simulink library "inp"  (Simulink 7.4)
settings: Solver=ode45  StartTime=0.0  StopTime=10.0  RelTol=1e-3
undefined symbols (not defined in the file): AINP_BrkPedalInterp_X_bar, C_TASK_10MS_S, ENUM_SHIFTER_D, ENUM_SHIFTER_N, ENUM_SHIFTER_P, ENUM_SHIFTER_R, KINP_BonnetCloseVehSpdThre_kph, KINP_EDUCoolantTempFilTm_s, KINP_EDUOilPressureFilTm_s, KINP_EDUOilTempFilTm_s, KINP_EDUSynchDisp_mm, KINP_EDUSynchPosnPWMDC_pct_LowerLimit, KINP_EDUSynchPosnPWMDC_pct_ovrdflg, KINP_EDUSynchPosnPWMDC_pct_ovrdval, KINP_EDUSynchPosnPWMDC_pct_UpperLimit, KINP_ShifterPosConfirmD_s, KINP_ShifterPosConfirmN_s, KINP_ShifterPosConfirmP_s, KINP_ShifterPosConfirmR_s, KINP_SingleAccPedalFltRateLim_pct, KINP_TMSpd2VehSpdSigNeg_rpm, KINP_TMSpd2VehSpdSigPos_rpm, KINP_ValidCheck_EDUSynchPosnPWMDC_dec, KINP_ValidCheck_EDUSynchPosnPWMDC_inc, KINP_ValidCheck_EDUSynchPosnPWMDC_lim, KINP_VehSpdSigKeepThres_kph, KPH2MPS, MIN2SEC, MINP_BrkPedalInterp_pct, MPS2KPH, PI, seat_version_control_block_callbacks, TIRE_RADIUS
libraries: inp_lib x166, hcu_lib x4, simulink x1
(part 2 of 9)

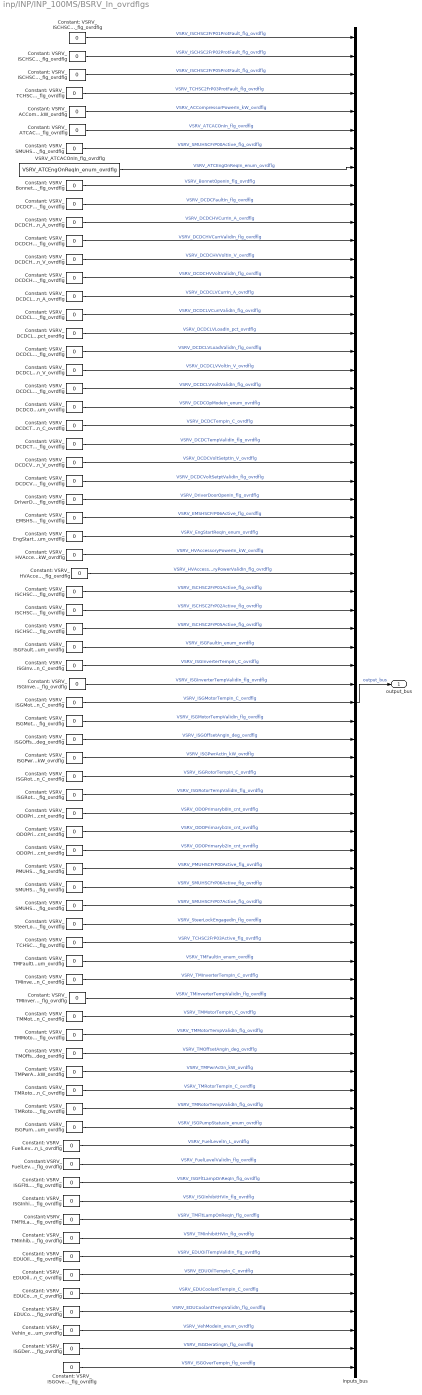
== system inp/INP/INP_100MS/BSRV_In_ovrdflgs ==
  Constant: VSRV_ACCompressorPowerIn_kW_ovrdflg : Constant  Value=0  OutDataTypeMode=boolean  OutDataTypeStr=boolean
  Constant: VSRV_ATCACOnIn_flg_ovrdflg : Constant  Value=0  OutDataTypeMode=boolean  OutDataTypeStr=boolean
  Constant: VSRV_BonnetOpenIn_flg_ovrdflg : Constant  Value=0  OutDataTypeMode=boolean  OutDataTypeStr=boolean
  Constant: VSRV_DCDCFaultIn_flg_ovrdflg : Constant  Value=0  OutDataTypeMode=boolean  OutDataTypeStr=boolean
  Constant: VSRV_DCDCHVCurrIn_A_ovrdflg : Constant  Value=0  OutDataTypeMode=boolean  OutDataTypeStr=boolean
  Constant: VSRV_DCDCHVCurrValidIn_flg_ovrdflg : Constant  Value=0  OutDataTypeMode=boolean  OutDataTypeStr=boolean
  Constant: VSRV_DCDCHVVoltIn_V_ovrdflg : Constant  Value=0  OutDataTypeMode=boolean  OutDataTypeStr=boolean
  Constant: VSRV_DCDCHVVoltValidIn_flg_ovrdflg : Constant  Value=0  OutDataTypeMode=boolean  OutDataTypeStr=boolean
  Constant: VSRV_DCDCLVCurrIn_A_ovrdflg : Constant  Value=0  OutDataTypeMode=boolean  OutDataTypeStr=boolean
  Constant: VSRV_DCDCLVCurrValidIn_flg_ovrdflg : Constant  Value=0  OutDataTypeMode=boolean  OutDataTypeStr=boolean
  Constant: VSRV_DCDCLVLoadIn_pct_ovrdflg : Constant  Value=0  OutDataTypeMode=boolean  OutDataTypeStr=boolean
  Constant: VSRV_DCDCLVLoadValidIn_flg_ovrdflg : Constant  Value=0  OutDataTypeMode=boolean  OutDataTypeStr=boolean
  Constant: VSRV_DCDCLVVoltIn_V_ovrdflg : Constant  Value=0  OutDataTypeMode=boolean  OutDataTypeStr=boolean
  Constant: VSRV_DCDCLVVoltValidIn_flg_ovrdflg : Constant  Value=0  OutDataTypeMode=boolean  OutDataTypeStr=boolean
  Constant: VSRV_DCDCOpModeIn_enum_ovrdflg : Constant  Value=0  OutDataTypeMode=boolean  OutDataTypeStr=boolean
  Constant: VSRV_DCDCTempIn_C_ovrdflg : Constant  Value=0  OutDataTypeMode=boolean  OutDataTypeStr=boolean
  Constant: VSRV_DCDCTempValidIn_flg_ovrdflg : Constant  Value=0  OutDataTypeMode=boolean  OutDataTypeStr=boolean
  Constant: VSRV_DCDCVoltSetptIn_V_ovrdflg : Constant  Value=0  OutDataTypeMode=boolean  OutDataTypeStr=boolean
  Constant: VSRV_DCDCVoltSetptValidIn_flg_ovrdflg : Constant  Value=0  OutDataTypeMode=boolean  OutDataTypeStr=boolean
  Constant: VSRV_DriverDoorOpenIn_flg_ovrdflg : Constant  Value=0  OutDataTypeMode=boolean  OutDataTypeStr=boolean
  Constant: VSRV_EDUCoolantTempIn_C_ovrdflg : Constant  Value=0  OutDataTypeMode=boolean  OutDataTypeStr=boolean
  Constant: VSRV_EDUCoolantTempValidIn_flg_ovrdflg : Constant  Value=0  OutDataTypeMode=boolean  OutDataTypeStr=boolean
  Constant: VSRV_EDUOilTempIn_C_ovrdflg : Constant  Value=0  OutDataTypeMode=boolean  OutDataTypeStr=boolean
  Constant: VSRV_EDUOilTempValidIn_flg_ovrdflg : Constant  Value=0  OutDataTypeMode=boolean  OutDataTypeStr=boolean
  Constant: VSRV_EMSHSCFrP06Active_flg_ovrdflg : Constant  Value=0  OutDataTypeMode=boolean  OutDataTypeStr=boolean
  Constant: VSRV_EngStartReqIn_enum_ovrdflg : Constant  Value=0  OutDataTypeMode=boolean  OutDataTypeStr=boolean
  Constant: VSRV_FuelLevelIn_L_ovrdflg : Constant  Value=0  OutDataTypeMode=boolean  OutDataTypeStr=boolean
  Constant: VSRV_HVAccessoryPowerIn_kW_ovrdflg : Constant  Value=0  OutDataTypeMode=boolean  OutDataTypeStr=boolean
  Constant: VSRV_HVAccessoryPowerValidIn_flg_ovrdflg : Constant  Value=0  OutDataTypeMode=boolean  OutDataTypeStr=boolean
  Constant: VSRV_ISCHSC2FrP01Active_flg_ovrdflg : Constant  Value=0  OutDataTypeMode=boolean  OutDataTypeStr=boolean
  Constant: VSRV_ISCHSC2FrP01ProtFault_flg_ovrdflg : Constant  Value=0  OutDataTypeMode=boolean  OutDataTypeStr=boolean
  Constant: VSRV_ISCHSC2FrP02Active_flg_ovrdflg : Constant  Value=0  OutDataTypeMode=boolean  OutDataTypeStr=boolean
  Constant: VSRV_ISCHSC2FrP02ProtFault_flg_ovrdflg : Constant  Value=0  OutDataTypeMode=boolean  OutDataTypeStr=boolean
  Constant: VSRV_ISCHSC2FrP05Active_flg_ovrdflg : Constant  Value=0  OutDataTypeMode=boolean  OutDataTypeStr=boolean
  Constant: VSRV_ISCHSC2FrP05ProtFault_flg_ovrdflg : Constant  Value=0  OutDataTypeMode=boolean  OutDataTypeStr=boolean
  Constant: VSRV_ISGDeratingIn_flg_ovrdflg : Constant  Value=0  OutDataTypeMode=boolean  OutDataTypeStr=boolean
  Constant: VSRV_ISGFaultIn_enum_ovrdflg : Constant  Value=0  OutDataTypeMode=boolean  OutDataTypeStr=boolean
  Constant: VSRV_ISGFltLampOnReqIn_flg_ovrdflg : Constant  Value=0  OutDataTypeMode=boolean  OutDataTypeStr=boolean
  Constant: VSRV_ISGInhibitHVIn_flg_ovrdflg : Constant  Value=0  OutDataTypeMode=boolean  OutDataTypeStr=boolean
  Constant: VSRV_ISGInverterTempIn_C_ovrdflg : Constant  Value=0  OutDataTypeMode=boolean  OutDataTypeStr=boolean
  Constant: VSRV_ISGInverterTempValidIn_flg_ovrdflg : Constant  Value=0  OutDataTypeMode=boolean  OutDataTypeStr=boolean
  Constant: VSRV_ISGMotorTempIn_C_ovrdflg : Constant  Value=0  OutDataTypeMode=boolean  OutDataTypeStr=boolean
  Constant: VSRV_ISGMotorTempValidIn_flg_ovrdflg : Constant  Value=0  OutDataTypeMode=boolean  OutDataTypeStr=boolean
  Constant: VSRV_ISGOffsetAngIn_deg_ovrdflg : Constant  Value=0  OutDataTypeMode=boolean  OutDataTypeStr=boolean
  Constant: VSRV_ISGOverTempIn_flg_ovrdflg : Constant  Value=0  OutDataTypeMode=boolean  OutDataTypeStr=boolean
  Constant: VSRV_ISGPumpStatusIn_enum_ovrdflg : Constant  Value=0  OutDataTypeMode=boolean  OutDataTypeStr=boolean
  Constant: VSRV_ISGPwrActIn_kW_ovrdflg : Constant  Value=0  OutDataTypeMode=boolean  OutDataTypeStr=boolean
  Constant: VSRV_ISGRotorTempIn_C_ovrdflg : Constant  Value=0  OutDataTypeMode=boolean  OutDataTypeStr=boolean
  Constant: VSRV_ISGRotorTempValidIn_flg_ovrdflg : Constant  Value=0  OutDataTypeMode=boolean  OutDataTypeStr=boolean
  Constant: VSRV_ODOPrimaryb0In_cnt_ovrdflg : Constant  Value=0  OutDataTypeMode=boolean  OutDataTypeStr=boolean
  Constant: VSRV_ODOPrimaryb1In_cnt_ovrdflg : Constant  Value=0  OutDataTypeMode=boolean  OutDataTypeStr=boolean
  Constant: VSRV_ODOPrimaryb2In_cnt_ovrdflg : Constant  Value=0  OutDataTypeMode=boolean  OutDataTypeStr=boolean
  Constant: VSRV_PMUHSCFrP00Active_flg_ovrdflg : Constant  Value=0  OutDataTypeMode=boolean  OutDataTypeStr=boolean
  Constant: VSRV_SMUHSCFrP00Active_flg_ovrdflg : Constant  Value=0  OutDataTypeMode=boolean  OutDataTypeStr=boolean
  Constant: VSRV_SMUHSCFrP06Active_flg_ovrdflg : Constant  Value=0  OutDataTypeMode=boolean  OutDataTypeStr=boolean
  Constant: VSRV_SMUHSCFrP07Active_flg_ovrdflg : Constant  Value=0  OutDataTypeMode=boolean  OutDataTypeStr=boolean
  Constant: VSRV_SteerLockEngagedIn_flg_ovrdflg : Constant  Value=0  OutDataTypeMode=boolean  OutDataTypeStr=boolean
  Constant: VSRV_TCHSC2FrP03Active_flg_ovrdflg : Constant  Value=0  OutDataTypeMode=boolean  OutDataTypeStr=boolean
  Constant: VSRV_TCHSC2FrP03ProtFault_flg_ovrdflg : Constant  Value=0  OutDataTypeMode=boolean  OutDataTypeStr=boolean
  Constant: VSRV_TMFaultIn_enum_ovrdflg : Constant  Value=0  OutDataTypeMode=boolean  OutDataTypeStr=boolean
  Constant: VSRV_TMInhibitHVIn_flg_ovrdflg : Constant  Value=0  OutDataTypeMode=boolean  OutDataTypeStr=boolean
  Constant: VSRV_TMInverterTempIn_C_ovrdflg : Constant  Value=0  OutDataTypeMode=boolean  OutDataTypeStr=boolean
  Constant: VSRV_TMInverterTempValidIn_flg_ovrdflg : Constant  Value=0  OutDataTypeMode=boolean  OutDataTypeStr=boolean
  Constant: VSRV_TMMotorTempIn_C_ovrdflg : Constant  Value=0  OutDataTypeMode=boolean  OutDataTypeStr=boolean
  Constant: VSRV_TMMotorTempValidIn_flg_ovrdflg : Constant  Value=0  OutDataTypeMode=boolean  OutDataTypeStr=boolean
  Constant: VSRV_TMOffsetAngIn_deg_ovrdflg : Constant  Value=0  OutDataTypeMode=boolean  OutDataTypeStr=boolean
  Constant: VSRV_TMPwrActIn_kW_ovrdflg : Constant  Value=0  OutDataTypeMode=boolean  OutDataTypeStr=boolean
  Constant: VSRV_TMRotorTempIn_C_ovrdflg : Constant  Value=0  OutDataTypeMode=boolean  OutDataTypeStr=boolean
  Constant: VSRV_TMRotorTempValidIn_flg_ovrdflg : Constant  Value=0  OutDataTypeMode=boolean  OutDataTypeStr=boolean
  Constant: VSRV_VehIn_enum_ovrdflg : Constant  Value=0  OutDataTypeMode=boolean  OutDataTypeStr=boolean
  Constant:VSRV_FuelLevelValidIn_flg_ovrdflg : Constant  Value=0  OutDataTypeMode=boolean  OutDataTypeStr=boolean
  Constant:VSRV_TMFltLampOnReqIn_flg_ovrdflg : Constant  Value=0  OutDataTypeMode=boolean  OutDataTypeStr=boolean
  VSRV_ATCACOnIn_flg_ovrdflg : DataStoreRead  DataStoreName=VSRV_ATCEngOnReqIn_enum_ovrdflg  SampleTime=-1
  inputs_bus : BusCreator  Inputs=73
  output_bus : Outport
  wires:
  Constant: VSRV_ISGOverTempIn_flg_ovrdflg/1 -> inputs_bus/73  "VSRV_ISGOverTempIn_flg_ovrdflg"
  Constant: VSRV_ISGDeratingIn_flg_ovrdflg/1 -> inputs_bus/72  "VSRV_ISGDeratingIn_flg_ovrdflg"
  Constant: VSRV_VehIn_enum_ovrdflg/1 -> inputs_bus/71  "VSRV_VehModeIn_enum_ovrdflg"
  Constant: VSRV_EDUCoolantTempValidIn_flg_ovrdflg/1 -> inputs_bus/70  "VSRV_EDUCoolantTempValidIn_flg_ovrdflg"
  Constant: VSRV_EDUCoolantTempIn_C_ovrdflg/1 -> inputs_bus/69  "VSRV_EDUCoolantTempIn_C_ovrdflg"
  Constant: VSRV_EDUOilTempIn_C_ovrdflg/1 -> inputs_bus/68  "VSRV_EDUOilTempIn_C_ovrdflg"
  Constant: VSRV_EDUOilTempValidIn_flg_ovrdflg/1 -> inputs_bus/67  "VSRV_EDUOilTempValidIn_flg_ovrdflg"
  Constant: VSRV_TMInhibitHVIn_flg_ovrdflg/1 -> inputs_bus/66  "VSRV_TMInhibitHVIn_flg_ovrdflg"
  Constant:VSRV_TMFltLampOnReqIn_flg_ovrdflg/1 -> inputs_bus/65  "VSRV_TMFltLampOnReqIn_flg_ovrdflg"
  Constant: VSRV_ISGInhibitHVIn_flg_ovrdflg/1 -> inputs_bus/64  "VSRV_ISGInhibitHVIn_flg_ovrdflg"
  Constant: VSRV_ISGFltLampOnReqIn_flg_ovrdflg/1 -> inputs_bus/63  "VSRV_ISGFltLampOnReqIn_flg_ovrdflg"
  Constant:VSRV_FuelLevelValidIn_flg_ovrdflg/1 -> inputs_bus/62  "VSRV_FuelLevelValidIn_flg_ovrdflg"
  Constant: VSRV_FuelLevelIn_L_ovrdflg/1 -> inputs_bus/61  "VSRV_FuelLevelIn_L_ovrdflg"
  Constant: VSRV_ISGPumpStatusIn_enum_ovrdflg/1 -> inputs_bus/60  "VSRV_ISGPumpStatusIn_enum_ovrdflg"
  Constant: VSRV_TMRotorTempValidIn_flg_ovrdflg/1 -> inputs_bus/59  "VSRV_TMRotorTempValidIn_flg_ovrdflg"
  Constant: VSRV_TMRotorTempIn_C_ovrdflg/1 -> inputs_bus/58  "VSRV_TMRotorTempIn_C_ovrdflg"
  Constant: VSRV_TMPwrActIn_kW_ovrdflg/1 -> inputs_bus/57  "VSRV_TMPwrActIn_kW_ovrdflg"
  Constant: VSRV_TMOffsetAngIn_deg_ovrdflg/1 -> inputs_bus/56  "VSRV_TMOffsetAngIn_deg_ovrdflg"
  Constant: VSRV_TMMotorTempValidIn_flg_ovrdflg/1 -> inputs_bus/55  "VSRV_TMMotorTempValidIn_flg_ovrdflg"
  Constant: VSRV_TMMotorTempIn_C_ovrdflg/1 -> inputs_bus/54  "VSRV_TMMotorTempIn_C_ovrdflg"
  Constant: VSRV_TMInverterTempValidIn_flg_ovrdflg/1 -> inputs_bus/53  "VSRV_TMInverterTempValidIn_flg_ovrdflg"
  Constant: VSRV_TMInverterTempIn_C_ovrdflg/1 -> inputs_bus/52  "VSRV_TMInverterTempIn_C_ovrdflg"
  Constant: VSRV_TMFaultIn_enum_ovrdflg/1 -> inputs_bus/51  "VSRV_TMFaultIn_enum_ovrdflg"
  Constant: VSRV_TCHSC2FrP03Active_flg_ovrdflg/1 -> inputs_bus/50  "VSRV_TCHSC2FrP03Active_flg_ovrdflg"
  Constant: VSRV_SteerLockEngagedIn_flg_ovrdflg/1 -> inputs_bus/49  "VSRV_SteerLockEngagedIn_flg_ovrdflg"
  Constant: VSRV_SMUHSCFrP07Active_flg_ovrdflg/1 -> inputs_bus/48  "VSRV_SMUHSCFrP07Active_flg_ovrdflg"
  Constant: VSRV_SMUHSCFrP06Active_flg_ovrdflg/1 -> inputs_bus/47  "VSRV_SMUHSCFrP06Active_flg_ovrdflg"
  Constant: VSRV_PMUHSCFrP00Active_flg_ovrdflg/1 -> inputs_bus/46  "VSRV_PMUHSCFrP00Active_flg_ovrdflg"
  Constant: VSRV_ODOPrimaryb2In_cnt_ovrdflg/1 -> inputs_bus/45  "VSRV_ODOPrimaryb2In_cnt_ovrdflg"
  Constant: VSRV_ODOPrimaryb1In_cnt_ovrdflg/1 -> inputs_bus/44  "VSRV_ODOPrimaryb1In_cnt_ovrdflg"
  Constant: VSRV_ODOPrimaryb0In_cnt_ovrdflg/1 -> inputs_bus/43  "VSRV_ODOPrimaryb0In_cnt_ovrdflg"
  Constant: VSRV_ISGRotorTempValidIn_flg_ovrdflg/1 -> inputs_bus/42  "VSRV_ISGRotorTempValidIn_flg_ovrdflg"
  Constant: VSRV_ISGRotorTempIn_C_ovrdflg/1 -> inputs_bus/41  "VSRV_ISGRotorTempIn_C_ovrdflg"
  Constant: VSRV_ISGPwrActIn_kW_ovrdflg/1 -> inputs_bus/40  "VSRV_ISGPwrActIn_kW_ovrdflg"
  Constant: VSRV_ISGOffsetAngIn_deg_ovrdflg/1 -> inputs_bus/39  "VSRV_ISGOffsetAngIn_deg_ovrdflg"
  Constant: VSRV_ISGMotorTempValidIn_flg_ovrdflg/1 -> inputs_bus/38  "VSRV_ISGMotorTempValidIn_flg_ovrdflg"
  Constant: VSRV_ISGMotorTempIn_C_ovrdflg/1 -> inputs_bus/37  "VSRV_ISGMotorTempIn_C_ovrdflg"
  Constant: VSRV_ISGInverterTempValidIn_flg_ovrdflg/1 -> inputs_bus/36  "VSRV_ISGInverterTempValidIn_flg_ovrdflg"
  Constant: VSRV_ISGInverterTempIn_C_ovrdflg/1 -> inputs_bus/35  "VSRV_ISGInverterTempIn_C_ovrdflg"
  Constant: VSRV_ISGFaultIn_enum_ovrdflg/1 -> inputs_bus/34  "VSRV_ISGFaultIn_enum_ovrdflg"
  Constant: VSRV_ISCHSC2FrP05Active_flg_ovrdflg/1 -> inputs_bus/33  "VSRV_ISCHSC2FrP05Active_flg_ovrdflg"
  Constant: VSRV_ISCHSC2FrP02Active_flg_ovrdflg/1 -> inputs_bus/32  "VSRV_ISCHSC2FrP02Active_flg_ovrdflg"
  Constant: VSRV_ISCHSC2FrP01Active_flg_ovrdflg/1 -> inputs_bus/31  "VSRV_ISCHSC2FrP01Active_flg_ovrdflg"
  Constant: VSRV_HVAccessoryPowerValidIn_flg_ovrdflg/1 -> inputs_bus/30  "VSRV_HVAccessoryPowerValidIn_flg_ovrdflg"
  Constant: VSRV_HVAccessoryPowerIn_kW_ovrdflg/1 -> inputs_bus/29  "VSRV_HVAccessoryPowerIn_kW_ovrdflg"
  Constant: VSRV_EngStartReqIn_enum_ovrdflg/1 -> inputs_bus/28  "VSRV_EngStartReqIn_enum_ovrdflg"
  Constant: VSRV_EMSHSCFrP06Active_flg_ovrdflg/1 -> inputs_bus/27  "VSRV_EMSHSCFrP06Active_flg_ovrdflg"
  Constant: VSRV_DriverDoorOpenIn_flg_ovrdflg/1 -> inputs_bus/26  "VSRV_DriverDoorOpenIn_flg_ovrdflg"
  Constant: VSRV_DCDCVoltSetptValidIn_flg_ovrdflg/1 -> inputs_bus/25  "VSRV_DCDCVoltSetptValidIn_flg_ovrdflg"
  Constant: VSRV_DCDCVoltSetptIn_V_ovrdflg/1 -> inputs_bus/24  "VSRV_DCDCVoltSetptIn_V_ovrdflg"
  Constant: VSRV_DCDCTempValidIn_flg_ovrdflg/1 -> inputs_bus/23  "VSRV_DCDCTempValidIn_flg_ovrdflg"
  Constant: VSRV_DCDCTempIn_C_ovrdflg/1 -> inputs_bus/22  "VSRV_DCDCTempIn_C_ovrdflg"
  Constant: VSRV_DCDCOpModeIn_enum_ovrdflg/1 -> inputs_bus/21  "VSRV_DCDCOpModeIn_enum_ovrdflg"
  Constant: VSRV_DCDCLVVoltValidIn_flg_ovrdflg/1 -> inputs_bus/20  "VSRV_DCDCLVVoltValidIn_flg_ovrdflg"
  Constant: VSRV_DCDCLVVoltIn_V_ovrdflg/1 -> inputs_bus/19  "VSRV_DCDCLVVoltIn_V_ovrdflg"
  Constant: VSRV_DCDCLVLoadValidIn_flg_ovrdflg/1 -> inputs_bus/18  "VSRV_DCDCLVLoadValidIn_flg_ovrdflg"
  Constant: VSRV_DCDCLVLoadIn_pct_ovrdflg/1 -> inputs_bus/17  "VSRV_DCDCLVLoadIn_pct_ovrdflg"
  Constant: VSRV_DCDCLVCurrValidIn_flg_ovrdflg/1 -> inputs_bus/16  "VSRV_DCDCLVCurrValidIn_flg_ovrdflg"
  Constant: VSRV_DCDCLVCurrIn_A_ovrdflg/1 -> inputs_bus/15  "VSRV_DCDCLVCurrIn_A_ovrdflg"
  Constant: VSRV_DCDCHVVoltValidIn_flg_ovrdflg/1 -> inputs_bus/14  "VSRV_DCDCHVVoltValidIn_flg_ovrdflg"
  Constant: VSRV_DCDCHVVoltIn_V_ovrdflg/1 -> inputs_bus/13  "VSRV_DCDCHVVoltIn_V_ovrdflg"
  Constant: VSRV_DCDCHVCurrValidIn_flg_ovrdflg/1 -> inputs_bus/12  "VSRV_DCDCHVCurrValidIn_flg_ovrdflg"
  Constant: VSRV_DCDCHVCurrIn_A_ovrdflg/1 -> inputs_bus/11  "VSRV_DCDCHVCurrIn_A_ovrdflg"
  Constant: VSRV_DCDCFaultIn_flg_ovrdflg/1 -> inputs_bus/10  "VSRV_DCDCFaultIn_flg_ovrdflg"
  Constant: VSRV_BonnetOpenIn_flg_ovrdflg/1 -> inputs_bus/9  "VSRV_BonnetOpenIn_flg_ovrdflg"
  VSRV_ATCACOnIn_flg_ovrdflg/1 -> inputs_bus/8  "VSRV_ATCEngOnReqIn_enum_ovrdflg"
  Constant: VSRV_SMUHSCFrP00Active_flg_ovrdflg/1 -> inputs_bus/7  "VSRV_SMUHSCFrP00Active_flg_ovrdflg"
  Constant: VSRV_ATCACOnIn_flg_ovrdflg/1 -> inputs_bus/6  "VSRV_ATCACOnIn_flg_ovrdflg"
  Constant: VSRV_ACCompressorPowerIn_kW_ovrdflg/1 -> inputs_bus/5  "VSRV_ACCompressorPowerIn_kW_ovrdflg"
  Constant: VSRV_TCHSC2FrP03ProtFault_flg_ovrdflg/1 -> inputs_bus/4  "VSRV_TCHSC2FrP03ProtFault_flg_ovrdflg"
  Constant: VSRV_ISCHSC2FrP05ProtFault_flg_ovrdflg/1 -> inputs_bus/3  "VSRV_ISCHSC2FrP05ProtFault_flg_ovrdflg"
  Constant: VSRV_ISCHSC2FrP02ProtFault_flg_ovrdflg/1 -> inputs_bus/2  "VSRV_ISCHSC2FrP02ProtFault_flg_ovrdflg"
  Constant: VSRV_ISCHSC2FrP01ProtFault_flg_ovrdflg/1 -> inputs_bus/1  "VSRV_ISCHSC2FrP01ProtFault_flg_ovrdflg"
  inputs_bus/1 -> output_bus/1  "output_bus"

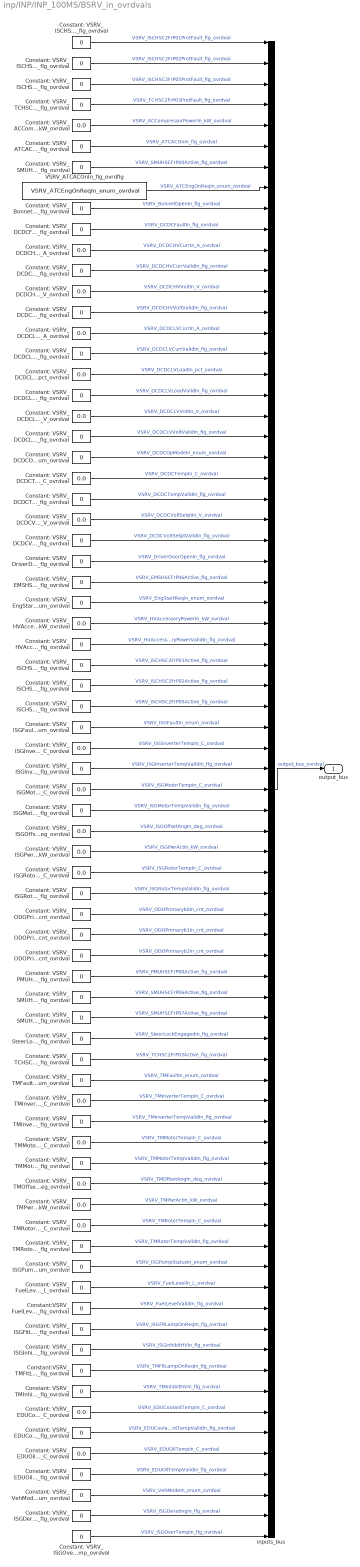
== system inp/INP/INP_100MS/BSRV_in_ovrdvals ==
  Constant: VSRV_ACCompressorPowerIn_kW_ovrdval : Constant  Value=0.0  OutDataTypeMode=single  OutDataTypeStr=single
  Constant: VSRV_ATCACOnIn_flg_ovrdval : Constant  Value=0  OutDataTypeMode=boolean  OutDataTypeStr=boolean
  Constant: VSRV_BonnetOpenIn_flg_ovrdval : Constant  Value=0  OutDataTypeMode=boolean  OutDataTypeStr=boolean
  Constant: VSRV_DCDCFaultIn_flg_ovrdval : Constant  Value=0  OutDataTypeMode=boolean  OutDataTypeStr=boolean
  Constant: VSRV_DCDCHVCurrIn_A_ovrdval : Constant  Value=0.0  OutDataTypeMode=single  OutDataTypeStr=single
  Constant: VSRV_DCDCHVCurrValidIn_flg_ovrdval : Constant  Value=0  OutDataTypeMode=boolean  OutDataTypeStr=boolean
  Constant: VSRV_DCDCHVVoltIn_V_ovrdval : Constant  Value=0.0  OutDataTypeMode=single  OutDataTypeStr=single
  Constant: VSRV_DCDCHVVoltValidIn_flg_ovrdval : Constant  Value=0  OutDataTypeMode=boolean  OutDataTypeStr=boolean
  Constant: VSRV_DCDCLVCurrIn_A_ovrdval : Constant  Value=0.0  OutDataTypeMode=single  OutDataTypeStr=single
  Constant: VSRV_DCDCLVCurrValidIn_flg_ovrdval : Constant  Value=0  OutDataTypeMode=boolean  OutDataTypeStr=boolean
  Constant: VSRV_DCDCLVLoadIn_pct_ovrdval : Constant  Value=0.0  OutDataTypeMode=single  OutDataTypeStr=single
  Constant: VSRV_DCDCLVLoadValidIn_flg_ovrdval : Constant  Value=0  OutDataTypeMode=boolean  OutDataTypeStr=boolean
  Constant: VSRV_DCDCLVVoltIn_V_ovrdval : Constant  Value=0.0  OutDataTypeMode=single  OutDataTypeStr=single
  Constant: VSRV_DCDCLVVoltValidIn_flg_ovrdval : Constant  Value=0  OutDataTypeMode=boolean  OutDataTypeStr=boolean
  Constant: VSRV_DCDCOpModeIn_enum_ovrdval : Constant  Value=0  OutDataTypeMode=uint8  OutDataTypeStr=uint8
  Constant: VSRV_DCDCTempIn_C_ovrdval : Constant  Value=0.0  OutDataTypeMode=single  OutDataTypeStr=single
  Constant: VSRV_DCDCTempValidIn_flg_ovrdval : Constant  Value=0  OutDataTypeMode=boolean  OutDataTypeStr=boolean
  Constant: VSRV_DCDCVoltSetptIn_V_ovrdval : Constant  Value=0.0  OutDataTypeMode=single  OutDataTypeStr=single
  Constant: VSRV_DCDCVoltSetptValidIn_flg_ovrdval : Constant  Value=0  OutDataTypeMode=boolean  OutDataTypeStr=boolean
  Constant: VSRV_DriverDoorOpenIn_flg_ovrdval : Constant  Value=0  OutDataTypeMode=boolean  OutDataTypeStr=boolean
  Constant: VSRV_EDUCoolantTempIn_C_ovrdval : Constant  Value=0.0  OutDataTypeMode=single  OutDataTypeStr=single
  Constant: VSRV_EDUCoolantTempValidIn_flg_ovrdval : Constant  Value=0  OutDataTypeMode=boolean  OutDataTypeStr=boolean
  Constant: VSRV_EDUOilTempIn_C_ovrdval : Constant  Value=0.0  OutDataTypeMode=single  OutDataTypeStr=single
  Constant: VSRV_EDUOilTempValidIn_flg_ovrdval : Constant  Value=0  OutDataTypeMode=boolean  OutDataTypeStr=boolean
  Constant: VSRV_EMSHSCFrP06Active_flg_ovrdval : Constant  Value=0  OutDataTypeMode=boolean  OutDataTypeStr=boolean
  Constant: VSRV_EngStartReqIn_enum_ovrdval : Constant  Value=0  OutDataTypeMode=uint8  OutDataTypeStr=uint8
  Constant: VSRV_FuelLevelIn_L_ovrdval : Constant  Value=0  OutDataTypeMode=single  OutDataTypeStr=single
  Constant: VSRV_HVAccessoryPowerIn_kW_ovrdval : Constant  Value=0.0  OutDataTypeMode=single  OutDataTypeStr=single
  Constant: VSRV_HVAccessoryPowerValidIn_flg_ovrdval : Constant  Value=0  OutDataTypeMode=boolean  OutDataTypeStr=boolean
  Constant: VSRV_ISCHSC2FrP01Active_flg_ovrdval : Constant  Value=0  OutDataTypeMode=boolean  OutDataTypeStr=boolean
  Constant: VSRV_ISCHSC2FrP01ProtFault_flg_ovrdval : Constant  Value=0  OutDataTypeMode=boolean  OutDataTypeStr=boolean
  Constant: VSRV_ISCHSC2FrP02Active_flg_ovrdval : Constant  Value=0  OutDataTypeMode=boolean  OutDataTypeStr=boolean
  Constant: VSRV_ISCHSC2FrP02ProtFault_flg_ovrdval : Constant  Value=0  OutDataTypeMode=boolean  OutDataTypeStr=boolean
  Constant: VSRV_ISCHSC2FrP05Active_flg_ovrdval : Constant  Value=0  OutDataTypeMode=boolean  OutDataTypeStr=boolean
  Constant: VSRV_ISCHSC2FrP05ProtFault_flg_ovrdval : Constant  Value=0  OutDataTypeMode=boolean  OutDataTypeStr=boolean
  Constant: VSRV_ISGDeratingIn_flg_ovrdval : Constant  Value=0  OutDataTypeMode=boolean  OutDataTypeStr=boolean
  Constant: VSRV_ISGFaultIn_enum_ovrdval : Constant  Value=0  OutDataTypeMode=uint8  OutDataTypeStr=uint8
  Constant: VSRV_ISGFltLampOnReqIn_flg_ovrdval : Constant  Value=0  OutDataTypeMode=boolean  OutDataTypeStr=boolean
  Constant: VSRV_ISGInhibitHVIn_flg_ovrdval : Constant  Value=0  OutDataTypeMode=boolean  OutDataTypeStr=boolean
  Constant: VSRV_ISGInverterTempIn_C_ovrdval : Constant  Value=0.0  OutDataTypeMode=single  OutDataTypeStr=single
  Constant: VSRV_ISGInverterTempValidIn_flg_ovrdval : Constant  Value=0  OutDataTypeMode=boolean  OutDataTypeStr=boolean
  Constant: VSRV_ISGMotorTempIn_C_ovrdval : Constant  Value=0.0  OutDataTypeMode=single  OutDataTypeStr=single
  Constant: VSRV_ISGMotorTempValidIn_flg_ovrdval : Constant  Value=0  OutDataTypeMode=boolean  OutDataTypeStr=boolean
  Constant: VSRV_ISGOffsetAngIn_deg_ovrdval : Constant  Value=0.0  OutDataTypeMode=single  OutDataTypeStr=single
  Constant: VSRV_ISGOverTemp_ovrdval : Constant  Value=0  OutDataTypeMode=boolean  OutDataTypeStr=boolean
  Constant: VSRV_ISGPumpStatusIn_enum_ovrdval : Constant  Value=0  OutDataTypeMode=uint8  OutDataTypeStr=uint8
  Constant: VSRV_ISGPwrActIn_kW_ovrdval : Constant  Value=0.0  OutDataTypeMode=single  OutDataTypeStr=single
  Constant: VSRV_ISGRotorTempIn_C_ovrdval : Constant  Value=0.0  OutDataTypeMode=single  OutDataTypeStr=single
  Constant: VSRV_ISGRotorTempValidIn_flg_ovrdval : Constant  Value=0  OutDataTypeMode=boolean  OutDataTypeStr=boolean
  Constant: VSRV_ODOPrimaryb0In_cnt_ovrdval : Constant  Value=0  OutDataTypeMode=uint8  OutDataTypeStr=uint8
  Constant: VSRV_ODOPrimaryb1In_cnt_ovrdval : Constant  Value=0  OutDataTypeMode=uint8  OutDataTypeStr=uint8
  Constant: VSRV_ODOPrimaryb2In_cnt_ovrdval : Constant  Value=0  OutDataTypeMode=uint8  OutDataTypeStr=uint8
  Constant: VSRV_PMUHSCFrP00Active_flg_ovrdval : Constant  Value=0  OutDataTypeMode=boolean  OutDataTypeStr=boolean
  Constant: VSRV_SMUHSCFrP00Active_flg_ovrdval : Constant  Value=0  OutDataTypeMode=boolean  OutDataTypeStr=boolean
  Constant: VSRV_SMUHSCFrP06Active_flg_ovrdval : Constant  Value=0  OutDataTypeMode=boolean  OutDataTypeStr=boolean
  Constant: VSRV_SMUHSCFrP07Active_flg_ovrdval : Constant  Value=0  OutDataTypeMode=boolean  OutDataTypeStr=boolean
  Constant: VSRV_SteerLockEngagedIn_flg_ovrdval : Constant  Value=0  OutDataTypeMode=boolean  OutDataTypeStr=boolean
  Constant: VSRV_TCHSC2FrP03Active_flg_ovrdval : Constant  Value=0  OutDataTypeMode=boolean  OutDataTypeStr=boolean
  Constant: VSRV_TCHSC2FrP03ProtFault_flg_ovrdval : Constant  Value=0  OutDataTypeMode=boolean  OutDataTypeStr=boolean
  Constant: VSRV_TMFaultIn_enum_ovrdval : Constant  Value=0  OutDataTypeMode=uint8  OutDataTypeStr=uint8
  Constant: VSRV_TMInhibitHVIn_flg_ovrdval : Constant  Value=0  OutDataTypeMode=boolean  OutDataTypeStr=boolean
  Constant: VSRV_TMInverterTempIn_C_ovrdval : Constant  Value=0.0  OutDataTypeMode=single  OutDataTypeStr=single
  Constant: VSRV_TMInverterTempValidIn_flg_ovrdval : Constant  Value=0  OutDataTypeMode=boolean  OutDataTypeStr=boolean
  Constant: VSRV_TMMotorTempIn_C_ovrdval : Constant  Value=0.0  OutDataTypeMode=single  OutDataTypeStr=single
  Constant: VSRV_TMMotorTempValidIn_flg_ovrdval : Constant  Value=0  OutDataTypeMode=boolean  OutDataTypeStr=boolean
  Constant: VSRV_TMOffsetAngIn_deg_ovrdval : Constant  Value=0.0  OutDataTypeMode=single  OutDataTypeStr=single
  Constant: VSRV_TMPwrActIn_kW_ovrdval : Constant  Value=0.0  OutDataTypeMode=single  OutDataTypeStr=single
  Constant: VSRV_TMRotorTempIn_C_ovrdval : Constant  Value=0.0  OutDataTypeMode=single  OutDataTypeStr=single
  Constant: VSRV_TMRotorTempValidIn_flg_ovrdval : Constant  Value=0  OutDataTypeMode=boolean  OutDataTypeStr=boolean
  Constant: VSRV_VehModeIn_enum_ovrdval : Constant  Value=0  OutDataTypeMode=uint8  OutDataTypeStr=uint8
  Constant:VSRV_FuelLevelValidIn_flg_ovrdval : Constant  Value=0  OutDataTypeMode=boolean  OutDataTypeStr=boolean
  Constant:VSRV_TMFltLampOnReqIn_flg_ovrdval : Constant  Value=0  OutDataTypeMode=boolean  OutDataTypeStr=boolean
  VSRV_ATCACOnIn_flg_ovrdflg : DataStoreRead  DataStoreName=VSRV_ATCEngOnReqIn_enum_ovrdval  SampleTime=-1
  inputs_bus : BusCreator  Inputs=73
  output_bus : Outport
  wires:
  Constant: VSRV_ISGOverTemp_ovrdval/1 -> inputs_bus/73  "VSRV_ISGOverTempIn_flg_ovrdval"
  Constant: VSRV_ISGDeratingIn_flg_ovrdval/1 -> inputs_bus/72  "VSRV_ISGDeratingIn_flg_ovrdval"
  Constant: VSRV_VehModeIn_enum_ovrdval/1 -> inputs_bus/71  "VSRV_VehModeIn_enum_ovrdval"
  Constant: VSRV_EDUOilTempValidIn_flg_ovrdval/1 -> inputs_bus/70  "VSRV_EDUOilTempValidIn_flg_ovrdval"
  Constant: VSRV_EDUOilTempIn_C_ovrdval/1 -> inputs_bus/69  "VSRV_EDUOilTempIn_C_ovrdval"
  Constant: VSRV_EDUCoolantTempValidIn_flg_ovrdval/1 -> inputs_bus/68  "VSRV_EDUCoolantTempValidIn_flg_ovrdval"
  Constant: VSRV_EDUCoolantTempIn_C_ovrdval/1 -> inputs_bus/67  "VSRV_EDUCoolantTempIn_C_ovrdval"
  Constant: VSRV_TMInhibitHVIn_flg_ovrdval/1 -> inputs_bus/66  "VSRV_TMInhibitHVIn_flg_ovrdval"
  Constant:VSRV_TMFltLampOnReqIn_flg_ovrdval/1 -> inputs_bus/65  "VSRV_TMFltLampOnReqIn_flg_ovrdval"
  Constant: VSRV_ISGInhibitHVIn_flg_ovrdval/1 -> inputs_bus/64  "VSRV_ISGInhibitHVIn_flg_ovrdval"
  Constant: VSRV_ISGFltLampOnReqIn_flg_ovrdval/1 -> inputs_bus/63  "VSRV_ISGFltLampOnReqIn_flg_ovrdval"
  Constant:VSRV_FuelLevelValidIn_flg_ovrdval/1 -> inputs_bus/62  "VSRV_FuelLevelValidIn_flg_ovrdval"
  Constant: VSRV_FuelLevelIn_L_ovrdval/1 -> inputs_bus/61  "VSRV_FuelLevelIn_L_ovrdval"
  Constant: VSRV_ISGPumpStatusIn_enum_ovrdval/1 -> inputs_bus/60  "VSRV_ISGPumpStatusIn_enum_ovrdval"
  Constant: VSRV_TMRotorTempValidIn_flg_ovrdval/1 -> inputs_bus/59  "VSRV_TMRotorTempValidIn_flg_ovrdval"
  Constant: VSRV_TMRotorTempIn_C_ovrdval/1 -> inputs_bus/58  "VSRV_TMRotorTempIn_C_ovrdval"
  Constant: VSRV_TMPwrActIn_kW_ovrdval/1 -> inputs_bus/57  "VSRV_TMPwrActIn_kW_ovrdval"
  Constant: VSRV_TMOffsetAngIn_deg_ovrdval/1 -> inputs_bus/56  "VSRV_TMOffsetAngIn_deg_ovrdval"
  Constant: VSRV_TMMotorTempValidIn_flg_ovrdval/1 -> inputs_bus/55  "VSRV_TMMotorTempValidIn_flg_ovrdval"
  Constant: VSRV_TMMotorTempIn_C_ovrdval/1 -> inputs_bus/54  "VSRV_TMMotorTempIn_C_ovrdval"
  Constant: VSRV_TMInverterTempValidIn_flg_ovrdval/1 -> inputs_bus/53  "VSRV_TMInverterTempValidIn_flg_ovrdval"
  Constant: VSRV_TMInverterTempIn_C_ovrdval/1 -> inputs_bus/52  "VSRV_TMInverterTempIn_C_ovrdval"
  Constant: VSRV_TMFaultIn_enum_ovrdval/1 -> inputs_bus/51  "VSRV_TMFaultIn_enum_ovrdval"
  Constant: VSRV_TCHSC2FrP03Active_flg_ovrdval/1 -> inputs_bus/50  "VSRV_TCHSC2FrP03Active_flg_ovrdval"
  Constant: VSRV_SteerLockEngagedIn_flg_ovrdval/1 -> inputs_bus/49  "VSRV_SteerLockEngagedIn_flg_ovrdval"
  Constant: VSRV_SMUHSCFrP07Active_flg_ovrdval/1 -> inputs_bus/48  "VSRV_SMUHSCFrP07Active_flg_ovrdval"
  Constant: VSRV_SMUHSCFrP06Active_flg_ovrdval/1 -> inputs_bus/47  "VSRV_SMUHSCFrP06Active_flg_ovrdval"
  Constant: VSRV_PMUHSCFrP00Active_flg_ovrdval/1 -> inputs_bus/46  "VSRV_PMUHSCFrP00Active_flg_ovrdval"
  Constant: VSRV_ODOPrimaryb2In_cnt_ovrdval/1 -> inputs_bus/45  "VSRV_ODOPrimaryb2In_cnt_ovrdval"
  Constant: VSRV_ODOPrimaryb1In_cnt_ovrdval/1 -> inputs_bus/44  "VSRV_ODOPrimaryb1In_cnt_ovrdval"
  Constant: VSRV_ODOPrimaryb0In_cnt_ovrdval/1 -> inputs_bus/43  "VSRV_ODOPrimaryb0In_cnt_ovrdval"
  Constant: VSRV_ISGRotorTempValidIn_flg_ovrdval/1 -> inputs_bus/42  "VSRV_ISGRotorTempValidIn_flg_ovrdval"
  Constant: VSRV_ISGRotorTempIn_C_ovrdval/1 -> inputs_bus/41  "VSRV_ISGRotorTempIn_C_ovrdval"
  Constant: VSRV_ISGPwrActIn_kW_ovrdval/1 -> inputs_bus/40  "VSRV_ISGPwrActIn_kW_ovrdval"
  Constant: VSRV_ISGOffsetAngIn_deg_ovrdval/1 -> inputs_bus/39  "VSRV_ISGOffsetAngIn_deg_ovrdval"
  Constant: VSRV_ISGMotorTempValidIn_flg_ovrdval/1 -> inputs_bus/38  "VSRV_ISGMotorTempValidIn_flg_ovrdval"
  Constant: VSRV_ISGMotorTempIn_C_ovrdval/1 -> inputs_bus/37  "VSRV_ISGMotorTempIn_C_ovrdval"
  Constant: VSRV_ISGInverterTempValidIn_flg_ovrdval/1 -> inputs_bus/36  "VSRV_ISGInverterTempValidIn_flg_ovrdval"
  Constant: VSRV_ISGInverterTempIn_C_ovrdval/1 -> inputs_bus/35  "VSRV_ISGInverterTempIn_C_ovrdval"
  Constant: VSRV_ISGFaultIn_enum_ovrdval/1 -> inputs_bus/34  "VSRV_ISGFaultIn_enum_ovrdval"
  Constant: VSRV_ISCHSC2FrP05Active_flg_ovrdval/1 -> inputs_bus/33  "VSRV_ISCHSC2FrP05Active_flg_ovrdval"
  Constant: VSRV_ISCHSC2FrP02Active_flg_ovrdval/1 -> inputs_bus/32  "VSRV_ISCHSC2FrP02Active_flg_ovrdval"
  Constant: VSRV_ISCHSC2FrP01Active_flg_ovrdval/1 -> inputs_bus/31  "VSRV_ISCHSC2FrP01Active_flg_ovrdval"
  Constant: VSRV_HVAccessoryPowerValidIn_flg_ovrdval/1 -> inputs_bus/30  "VSRV_HVAccessoryPowerValidIn_flg_ovrdval"
  Constant: VSRV_HVAccessoryPowerIn_kW_ovrdval/1 -> inputs_bus/29  "VSRV_HVAccessoryPowerIn_kW_ovrdval"
  Constant: VSRV_EngStartReqIn_enum_ovrdval/1 -> inputs_bus/28  "VSRV_EngStartReqIn_enum_ovrdval"
  Constant: VSRV_EMSHSCFrP06Active_flg_ovrdval/1 -> inputs_bus/27  "VSRV_EMSHSCFrP06Active_flg_ovrdval"
  Constant: VSRV_DriverDoorOpenIn_flg_ovrdval/1 -> inputs_bus/26  "VSRV_DriverDoorOpenIn_flg_ovrdval"
  Constant: VSRV_DCDCVoltSetptValidIn_flg_ovrdval/1 -> inputs_bus/25  "VSRV_DCDCVoltSetptValidIn_flg_ovrdval"
  Constant: VSRV_DCDCVoltSetptIn_V_ovrdval/1 -> inputs_bus/24  "VSRV_DCDCVoltSetptIn_V_ovrdval"
  Constant: VSRV_DCDCTempValidIn_flg_ovrdval/1 -> inputs_bus/23  "VSRV_DCDCTempValidIn_flg_ovrdval"
  Constant: VSRV_DCDCTempIn_C_ovrdval/1 -> inputs_bus/22  "VSRV_DCDCTempIn_C_ovrdval"
  Constant: VSRV_DCDCOpModeIn_enum_ovrdval/1 -> inputs_bus/21  "VSRV_DCDCOpModeIn_enum_ovrdval"
  Constant: VSRV_DCDCLVVoltValidIn_flg_ovrdval/1 -> inputs_bus/20  "VSRV_DCDCLVVoltValidIn_flg_ovrdval"
  Constant: VSRV_DCDCLVVoltIn_V_ovrdval/1 -> inputs_bus/19  "VSRV_DCDCLVVoltIn_V_ovrdval"
  Constant: VSRV_DCDCLVLoadValidIn_flg_ovrdval/1 -> inputs_bus/18  "VSRV_DCDCLVLoadValidIn_flg_ovrdval"
  Constant: VSRV_DCDCLVLoadIn_pct_ovrdval/1 -> inputs_bus/17  "VSRV_DCDCLVLoadIn_pct_ovrdval"
  Constant: VSRV_DCDCLVCurrValidIn_flg_ovrdval/1 -> inputs_bus/16  "VSRV_DCDCLVCurrValidIn_flg_ovrdval"
  Constant: VSRV_DCDCLVCurrIn_A_ovrdval/1 -> inputs_bus/15  "VSRV_DCDCLVCurrIn_A_ovrdval"
  Constant: VSRV_DCDCHVVoltValidIn_flg_ovrdval/1 -> inputs_bus/14  "VSRV_DCDCHVVoltValidIn_flg_ovrdval"
  Constant: VSRV_DCDCHVVoltIn_V_ovrdval/1 -> inputs_bus/13  "VSRV_DCDCHVVoltIn_V_ovrdval"
  Constant: VSRV_DCDCHVCurrValidIn_flg_ovrdval/1 -> inputs_bus/12  "VSRV_DCDCHVCurrValidIn_flg_ovrdval"
  Constant: VSRV_DCDCHVCurrIn_A_ovrdval/1 -> inputs_bus/11  "VSRV_DCDCHVCurrIn_A_ovrdval"
  Constant: VSRV_DCDCFaultIn_flg_ovrdval/1 -> inputs_bus/10  "VSRV_DCDCFaultIn_flg_ovrdval"
  Constant: VSRV_BonnetOpenIn_flg_ovrdval/1 -> inputs_bus/9  "VSRV_BonnetOpenIn_flg_ovrdval"
  VSRV_ATCACOnIn_flg_ovrdflg/1 -> inputs_bus/8  "VSRV_ATCEngOnReqIn_enum_ovrdval"
  Constant: VSRV_SMUHSCFrP00Active_flg_ovrdval/1 -> inputs_bus/7  "VSRV_SMUHSCFrP00Active_flg_ovrdval"
  Constant: VSRV_ATCACOnIn_flg_ovrdval/1 -> inputs_bus/6  "VSRV_ATCACOnIn_flg_ovrdval"
  Constant: VSRV_ACCompressorPowerIn_kW_ovrdval/1 -> inputs_bus/5  "VSRV_ACCompressorPowerIn_kW_ovrdval"
  Constant: VSRV_TCHSC2FrP03ProtFault_flg_ovrdval/1 -> inputs_bus/4  "VSRV_TCHSC2FrP03ProtFault_flg_ovrdval"
  Constant: VSRV_ISCHSC2FrP05ProtFault_flg_ovrdval/1 -> inputs_bus/3  "VSRV_ISCHSC2FrP05ProtFault_flg_ovrdval"
  Constant: VSRV_ISCHSC2FrP02ProtFault_flg_ovrdval/1 -> inputs_bus/2  "VSRV_ISCHSC2FrP02ProtFault_flg_ovrdval"
  Constant: VSRV_ISCHSC2FrP01ProtFault_flg_ovrdval/1 -> inputs_bus/1  "VSRV_ISCHSC2FrP01ProtFault_flg_ovrdval"
  inputs_bus/1 -> output_bus/1  "output_bus_ovrdval"

== system inp/INP/INP_100MS/HW_HCU_100ms ==
  BHAL_IN_100ms : Inport
  BSRV_In_ovrdflgs : Inport  Port=2
  BSRV_In_ovrdvals : Inport  Port=3
  Bus Creator : BusCreator  Inputs=5
  Bus Selector1 : BusSelector  OutputSignals=VHAL_VehModeIn_enum
  Bus Selector10 : BusSelector  OutputSignals=VSRV_EDUOilTempIn_C_ovrdval
  Bus Selector11 : BusSelector  OutputSignals=VSRV_EDUCoolantTempIn_C_ovrdval
  Bus Selector12 : BusSelector  OutputSignals=VSRV_EDUCoolantTempIn_C_ovrdflg
  Bus Selector13 : BusSelector  OutputSignals=VSRV_EDUOilTempIn_C_ovrdflg
  Bus Selector2 : BusSelector  OutputSignals=VHAL_EDUCoolantTempIn_C
  Bus Selector38 : BusSelector  OutputSignals=VHAL_EDUOilTempValidIn_flg
  Bus Selector39 : BusSelector  OutputSignals=VHAL_EDUCoolantTempValidIn_flg
  Bus Selector4 : BusSelector  OutputSignals=VSRV_VehModeIn_enum_ovrdval
  Bus Selector5 : BusSelector  OutputSignals=VSRV_VehModeIn_enum_ovrdflg
  Bus Selector6 : BusSelector  OutputSignals=VHAL_EDUOilTempIn_C
  Subsys VINP_EDUCoolantTemp_C : inp_lib/valid_sat_ovrd  SystemSampleTime=-1  cal_ovrdflg=KINP_EDUCoolantTemp_C_ovrdflg  cal_ovrdval=KINP_EDUCoolantTemp_C_ovrdval  lim=KINP_ValidCheck_EDUCoolantTemp_lim  inc=KINP_ValidCheck_EDUCoolantTemp_inc  dec=KINP_ValidCheck_EDUCoolantTemp_dec  default=KINP_EDUCoolantTempDefault_C  hi=KINP_EDUCoolantTemp_C_UpperLimit  lo=KINP_EDUCoolantTemp_C_LowerLimit
  Subsys VINP_EDUOilTemp_C : inp_lib/valid_sat_ovrd  SystemSampleTime=-1  cal_ovrdflg=KINP_EDUOilTemp_C_ovrdflg  cal_ovrdval=KINP_EDUOilTemp_C_ovrdval  lim=KINP_ValidCheck_EDUOilTemp_lim  inc=KINP_ValidCheck_EDUOilTemp_inc  dec=KINP_ValidCheck_EDUOilTemp_dec  default=KINP_EDUOilTempDefault_C  hi=KINP_EDUOilTemp_C_UpperLimit  lo=KINP_EDUOilTemp_C_LowerLimit
  Subsys VINP_VehMode_enum : inp_lib/override  SystemSampleTime=-1  cal_ovrdflg=KINP_VehMode_enum_ovrdflg  cal_ovrdval=KINP_VehMode_enum_ovrdval
  filter : Subsystem
      settings: RTWSystemCode=Inline
  filter1 : Subsystem
      settings: RTWSystemCode=Inline
  BINP_HW_HCU_100ms : Outport
  wires:
  filter1/1(VINP_EDUOilTemp_C) -> Bus Creator/3  "VINP_EDUOilTemp_C"
  filter/1(VINP_EDUCoolantTemp_C) -> Bus Creator/1  "VINP_EDUCoolantTemp_C"
  [BSRV_In_ovrdvals] -> Bus Selector4/1
  [BSRV_In_ovrdflgs] -> Bus Selector5/1
  Bus Creator/1 -> BINP_HW_HCU_100ms/1  "BINP_HW_HCU_100ms"
  BSRV_In_ovrdflgs/1 -> [BSRV_In_ovrdflgs]
  BSRV_In_ovrdvals/1 -> [BSRV_In_ovrdvals]
  [BSRV_In_ovrdflgs] -> Bus Selector12/1
  [BSRV_In_ovrdvals] -> Bus Selector11/1
  BHAL_IN_100ms/1 -> Bus Selector1/1, Bus Selector38/1, Bus Selector6/1, Bus Selector39/1, Bus Selector2/1
  [BSRV_In_ovrdflgs] -> Bus Selector13/1
  [BSRV_In_ovrdvals] -> Bus Selector10/1
  Bus Selector2/1 -> Subsys VINP_EDUCoolantTemp_C/1  "<VHAL_EDUCoolantTempIn_C>"
  Bus Selector39/1 -> Subsys VINP_EDUCoolantTemp_C/2  "<VHAL_EDUCoolantTempValidIn_flg>"
  Bus Selector12/1 -> Subsys VINP_EDUCoolantTemp_C/3  "<VSRV_EDUCoolantTempIn_C_ovrdflg>"
  Bus Selector11/1 -> Subsys VINP_EDUCoolantTemp_C/4  "<VSRV_EDUCoolantTempIn_C_ovrdval>"
  Subsys VINP_EDUCoolantTemp_C/1 -> filter/1(VINP_EDUCoolantTempRaw_C)  "VINP_EDUCoolantTempRaw_C"
  Subsys VINP_EDUCoolantTemp_C/2 -> Bus Creator/2  "VINP_EDUCoolantTempValid_flg"
  Bus Selector6/1 -> Subsys VINP_EDUOilTemp_C/1  "<VHAL_EDUOilTempIn_C>"
  Bus Selector38/1 -> Subsys VINP_EDUOilTemp_C/2  "<VHAL_EDUOilTempValidIn_flg>"
  Bus Selector13/1 -> Subsys VINP_EDUOilTemp_C/3  "<VSRV_EDUOilTempIn_C_ovrdflg>"
  Bus Selector10/1 -> Subsys VINP_EDUOilTemp_C/4  "<VSRV_EDUOilTempIn_C_ovrdval>"
  Subsys VINP_EDUOilTemp_C/1 -> filter1/1(VINP_EDUOilTempRaw_C)  "VINP_EDUOilTempRaw_C"
  Subsys VINP_EDUOilTemp_C/2 -> Bus Creator/4  "VINP_EDUOilTempValid_flg"
  Bus Selector1/1 -> Subsys VINP_VehMode_enum/1  "<VHAL_VehModeIn_enum>"
  Bus Selector5/1 -> Subsys VINP_VehMode_enum/2  "<VSRV_VehModeIn_enum_ovrdflg>"
  Bus Selector4/1 -> Subsys VINP_VehMode_enum/3  "<VSRV_VehModeIn_enum_ovrdval>"
  Subsys VINP_VehMode_enum/1 -> Bus Creator/5  "VINP_VehMode_enum"

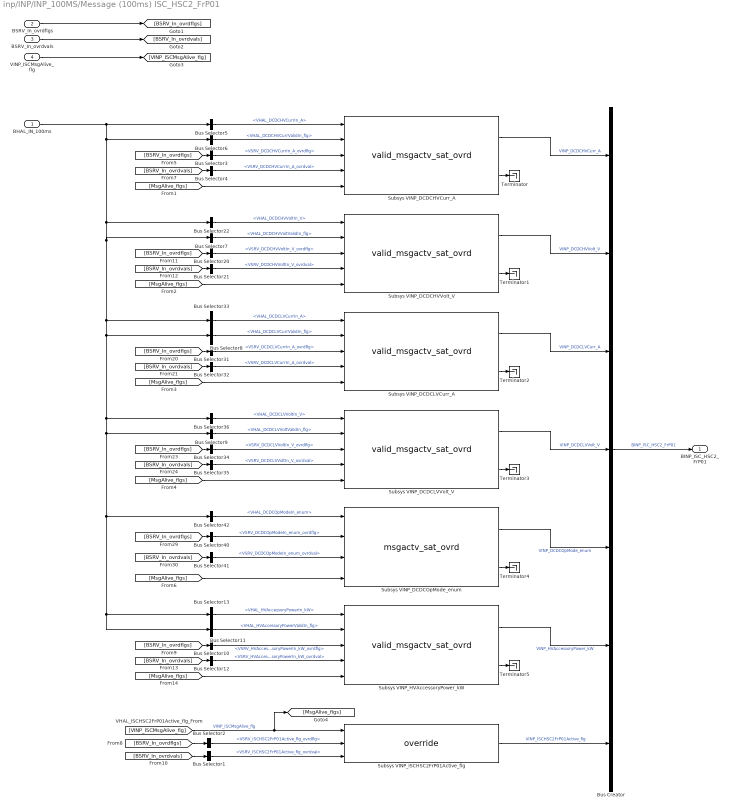
== system inp/INP/INP_100MS/Message (100ms) ISC_HSC2_FrP01 ==
  BHAL_IN_100ms : Inport
  BSRV_In_ovrdflgs : Inport  Port=2
  BSRV_In_ovrdvals : Inport  Port=3
  VINP_ISCMsgAlive_flg : Inport  Port=4
  Bus Creator : BusCreator  Inputs=7
  Bus Selector1 : BusSelector  OutputSignals=VSRV_ISCHSC2FrP01Active_flg_ovrdval
  Bus Selector10 : BusSelector  OutputSignals=VSRV_HVAccessoryPowerIn_kW_ovrdflg
  Bus Selector11 : BusSelector  OutputSignals=VHAL_HVAccessoryPowerValidIn_flg
  Bus Selector12 : BusSelector  OutputSignals=VSRV_HVAccessoryPowerIn_kW_ovrdval
  Bus Selector13 : BusSelector  OutputSignals=VHAL_HVAccessoryPowerIn_kW
  Bus Selector2 : BusSelector  OutputSignals=VSRV_ISCHSC2FrP01Active_flg_ovrdflg
  Bus Selector20 : BusSelector  OutputSignals=VSRV_DCDCHVVoltIn_V_ovrdflg
  Bus Selector21 : BusSelector  OutputSignals=VSRV_DCDCHVVoltIn_V_ovrdval
  Bus Selector22 : BusSelector  OutputSignals=VHAL_DCDCHVVoltIn_V
  Bus Selector3 : BusSelector  OutputSignals=VSRV_DCDCHVCurrIn_A_ovrdflg
  Bus Selector31 : BusSelector  OutputSignals=VSRV_DCDCLVCurrIn_A_ovrdflg
  Bus Selector32 : BusSelector  OutputSignals=VSRV_DCDCLVCurrIn_A_ovrdval
  Bus Selector33 : BusSelector  OutputSignals=VHAL_DCDCLVCurrIn_A
  Bus Selector34 : BusSelector  OutputSignals=VSRV_DCDCLVVoltIn_V_ovrdflg
  Bus Selector35 : BusSelector  OutputSignals=VSRV_DCDCLVVoltIn_V_ovrdval
  Bus Selector36 : BusSelector  OutputSignals=VHAL_DCDCLVVoltIn_V
  Bus Selector4 : BusSelector  OutputSignals=VSRV_DCDCHVCurrIn_A_ovrdval
  Bus Selector40 : BusSelector  OutputSignals=VSRV_DCDCOpModeIn_enum_ovrdflg
  Bus Selector41 : BusSelector  OutputSignals=VSRV_DCDCOpModeIn_enum_ovrdval
  Bus Selector42 : BusSelector  OutputSignals=VHAL_DCDCOpModeIn_enum
  Bus Selector5 : BusSelector  OutputSignals=VHAL_DCDCHVCurrIn_A
  Bus Selector6 : BusSelector  OutputSignals=VHAL_DCDCHVCurrValidIn_flg
  Bus Selector7 : BusSelector  OutputSignals=VHAL_DCDCHVVoltValidIn_flg
  Bus Selector8 : BusSelector  OutputSignals=VHAL_DCDCLVCurrValidIn_flg
  Bus Selector9 : BusSelector  OutputSignals=VHAL_DCDCLVVoltValidIn_flg
  Subsys VINP_DCDCHVCurr_A : inp_lib/valid_msgactv_sat_ovrd  SystemSampleTime=-1  cal_ovrdflg=KINP_DCDCHVCurr_A_ovrdflg  cal_ovrdval=KINP_DCDCHVCurr_A_ovrdval  lim=KINP_ValidCheck_DCDCHVCurr_lim  inc=KINP_ValidCheck_DCDCHVCurr_inc  dec=KINP_ValidCheck_DCDCHVCurr_dec  default=KINP_DCDCHVCurrDefault_A  hi=KINP_DCDCHVCurr_A_Max  lo=KINP_DCDCHVCurr_A_Min
  Subsys VINP_DCDCHVVolt_V : inp_lib/valid_msgactv_sat_ovrd  SystemSampleTime=-1  cal_ovrdflg=KINP_DCDCHVVolt_V_ovrdflg  cal_ovrdval=KINP_DCDCHVVolt_V_ovrdval  lim=KINP_ValidCheck_DCDCHVVolt_lim  inc=KINP_ValidCheck_DCDCHVVolt_inc  dec=KINP_ValidCheck_DCDCHVVolt_dec  default=KINP_DCDCHVVoltDefault_V  hi=KINP_DCDCHVVolt_V_Max  lo=KINP_DCDCHVVolt_V_Min
  Subsys VINP_DCDCLVCurr_A : inp_lib/valid_msgactv_sat_ovrd  SystemSampleTime=-1  cal_ovrdflg=KINP_DCDCLVCurr_A_ovrdflg  cal_ovrdval=KINP_DCDCLVCurr_A_ovrdval  lim=KINP_ValidCheck_DCDCLVCurr_lim  inc=KINP_ValidCheck_DCDCLVCurr_inc  dec=KINP_ValidCheck_DCDCLVCurr_dec  default=KINP_DCDCLVCurrDefault_A  hi=KINP_DCDCLVCurr_A_Max  lo=KINP_DCDCLVCurr_A_Min
  Subsys VINP_DCDCLVVolt_V : inp_lib/valid_msgactv_sat_ovrd  SystemSampleTime=-1  cal_ovrdflg=KINP_DCDCLVVolt_V_ovrdflg  cal_ovrdval=KINP_DCDCLVVolt_V_ovrdval  lim=KINP_ValidCheck_DCDCLVVolt_lim  inc=KINP_ValidCheck_DCDCLVVolt_inc  dec=KINP_ValidCheck_DCDCLVVolt_dec  default=KINP_DCDCLVVoltDefault_V  hi=KINP_DCDCLVVolt_V_Max  lo=KINP_DCDCLVVolt_V_Min
  Subsys VINP_DCDCOpMode_enum : inp_lib/msgactv_sat_ovrd  SystemSampleTime=-1  cal_ovrdflg=KINP_DCDCOpMode_enum_ovrdflg  cal_ovrdval=KINP_DCDCOpMode_enum_ovrdval  default=KINP_DCDCOpModeDefault_enum  hi=KINP_DCDCOpMode_enum_Max  lo=KINP_DCDCOpMode_enum_Min
  Subsys VINP_HVAccessoryPower_kW : inp_lib/valid_msgactv_sat_ovrd  SystemSampleTime=-1  cal_ovrdflg=KINP_HVAccessoryPower_kW_ovrdflg  cal_ovrdval=KINP_HVAccessoryPower_kW_ovrdval  lim=KINP_ValidCheck_HVAccessoryPower_lim  inc=KINP_ValidCheck_HVAccessoryPower_inc  dec=KINP_ValidCheck_HVAccessoryPower_dec  default=KINP_HVAccessoryPowerDefault_kW  hi=KINP_HVAccessoryPower_kW_Max  lo=KINP_HVAccessoryPower_kW_Min
  Subsys VINP_ISCHSC2FrP01Active_flg : inp_lib/override  SystemSampleTime=-1  cal_ovrdflg=KINP_ISCHSC2FrP01Active_ovrdflg  cal_ovrdval=KINP_ISCHSC2FrP01Active_flg_ovrdval
  Terminator{,1..5} (6 alike) : Terminator
  BINP_ISC_HSC2_FrP01 : Outport
  wires:
  [BSRV_In_ovrdvals] -> Bus Selector41/1
  [BSRV_In_ovrdflgs] -> Bus Selector40/1
  [BSRV_In_ovrdvals] -> Bus Selector35/1
  [BSRV_In_ovrdflgs] -> Bus Selector34/1
  [BSRV_In_ovrdvals] -> Bus Selector32/1
  [BSRV_In_ovrdflgs] -> Bus Selector31/1
  [BSRV_In_ovrdvals] -> Bus Selector21/1
  [BSRV_In_ovrdflgs] -> Bus Selector20/1
  [BSRV_In_ovrdvals] -> Bus Selector4/1
  [BSRV_In_ovrdflgs] -> Bus Selector3/1
  BHAL_IN_100ms/1 -> Bus Selector6/1, Bus Selector7/1, Bus Selector8/1, Bus Selector9/1, Bus Selector42/1, Bus Selector13/1, Bus Selector11/1, Bus Selector36/1, Bus Selector33/1, Bus Selector22/1, Bus Selector5/1
  VINP_ISCMsgAlive_flg/1 -> [VINP_ISCMsgAlive_flg]
  BSRV_In_ovrdflgs/1 -> [BSRV_In_ovrdflgs]
  BSRV_In_ovrdvals/1 -> [BSRV_In_ovrdvals]
  Bus Creator/1 -> BINP_ISC_HSC2_FrP01/1  "BINP_ISC_HSC2_FrP01"
  [BSRV_In_ovrdvals] -> Bus Selector12/1
  [BSRV_In_ovrdflgs] -> Bus Selector10/1
  [BSRV_In_ovrdvals] -> Bus Selector1/1
  [BSRV_In_ovrdflgs] -> Bus Selector2/1
  Bus Selector5/1 -> Subsys VINP_DCDCHVCurr_A/1  "<VHAL_DCDCHVCurrIn_A>"
  Bus Selector6/1 -> Subsys VINP_DCDCHVCurr_A/2  "<VHAL_DCDCHVCurrValidIn_flg>"
  Bus Selector3/1 -> Subsys VINP_DCDCHVCurr_A/3  "<VSRV_DCDCHVCurrIn_A_ovrdflg>"
  Bus Selector4/1 -> Subsys VINP_DCDCHVCurr_A/4  "<VSRV_DCDCHVCurrIn_A_ovrdval>"
  [MsgAlive_flgs] -> Subsys VINP_DCDCHVCurr_A/5
  Subsys VINP_DCDCHVCurr_A/1 -> Bus Creator/1  "VINP_DCDCHVCurr_A"
  Subsys VINP_DCDCHVCurr_A/2 -> Terminator/1
  Bus Selector22/1 -> Subsys VINP_DCDCHVVolt_V/1  "<VHAL_DCDCHVVoltIn_V>"
  Bus Selector7/1 -> Subsys VINP_DCDCHVVolt_V/2  "<VHAL_DCDCHVVoltValidIn_flg>"
  Bus Selector20/1 -> Subsys VINP_DCDCHVVolt_V/3  "<VSRV_DCDCHVVoltIn_V_ovrdflg>"
  Bus Selector21/1 -> Subsys VINP_DCDCHVVolt_V/4  "<VSRV_DCDCHVVoltIn_V_ovrdval>"
  [MsgAlive_flgs] -> Subsys VINP_DCDCHVVolt_V/5
  Subsys VINP_DCDCHVVolt_V/1 -> Bus Creator/2  "VINP_DCDCHVVolt_V"
  Subsys VINP_DCDCHVVolt_V/2 -> Terminator1/1
  Bus Selector33/1 -> Subsys VINP_DCDCLVCurr_A/1  "<VHAL_DCDCLVCurrIn_A>"
  Bus Selector8/1 -> Subsys VINP_DCDCLVCurr_A/2  "<VHAL_DCDCLVCurrValidIn_flg>"
  Bus Selector31/1 -> Subsys VINP_DCDCLVCurr_A/3  "<VSRV_DCDCLVCurrIn_A_ovrdflg>"
  Bus Selector32/1 -> Subsys VINP_DCDCLVCurr_A/4  "<VSRV_DCDCLVCurrIn_A_ovrdval>"
  [MsgAlive_flgs] -> Subsys VINP_DCDCLVCurr_A/5
  Subsys VINP_DCDCLVCurr_A/1 -> Bus Creator/3  "VINP_DCDCLVCurr_A"
  Subsys VINP_DCDCLVCurr_A/2 -> Terminator2/1
  Bus Selector36/1 -> Subsys VINP_DCDCLVVolt_V/1  "<VHAL_DCDCLVVoltIn_V>"
  Bus Selector9/1 -> Subsys VINP_DCDCLVVolt_V/2  "<VHAL_DCDCLVVoltValidIn_flg>"
  Bus Selector34/1 -> Subsys VINP_DCDCLVVolt_V/3  "<VSRV_DCDCLVVoltIn_V_ovrdflg>"
  Bus Selector35/1 -> Subsys VINP_DCDCLVVolt_V/4  "<VSRV_DCDCLVVoltIn_V_ovrdval>"
  [MsgAlive_flgs] -> Subsys VINP_DCDCLVVolt_V/5
  Subsys VINP_DCDCLVVolt_V/1 -> Bus Creator/4  "VINP_DCDCLVVolt_V"
  Subsys VINP_DCDCLVVolt_V/2 -> Terminator3/1
  Bus Selector42/1 -> Subsys VINP_DCDCOpMode_enum/1  "<VHAL_DCDCOpModeIn_enum>"
  Bus Selector40/1 -> Subsys VINP_DCDCOpMode_enum/2  "<VSRV_DCDCOpModeIn_enum_ovrdflg>"
  Bus Selector41/1 -> Subsys VINP_DCDCOpMode_enum/3  "<VSRV_DCDCOpModeIn_enum_ovrdval>"
  [MsgAlive_flgs] -> Subsys VINP_DCDCOpMode_enum/4
  Subsys VINP_DCDCOpMode_enum/1 -> Bus Creator/5  "VINP_DCDCOpMode_enum"
  Subsys VINP_DCDCOpMode_enum/2 -> Terminator4/1
  Bus Selector13/1 -> Subsys VINP_HVAccessoryPower_kW/1  "<VHAL_HVAccessoryPowerIn_kW>"
  Bus Selector11/1 -> Subsys VINP_HVAccessoryPower_kW/2  "<VHAL_HVAccessoryPowerValidIn_flg>"
  Bus Selector10/1 -> Subsys VINP_HVAccessoryPower_kW/3  "<VSRV_HVAccessoryPowerIn_kW_ovrdflg>"
  Bus Selector12/1 -> Subsys VINP_HVAccessoryPower_kW/4  "<VSRV_HVAccessoryPowerIn_kW_ovrdval>"
  [MsgAlive_flgs] -> Subsys VINP_HVAccessoryPower_kW/5
  Subsys VINP_HVAccessoryPower_kW/1 -> Bus Creator/6  "VINP_HVAccessoryPower_kW"
  Subsys VINP_HVAccessoryPower_kW/2 -> Terminator5/1
  Bus Selector2/1 -> Subsys VINP_ISCHSC2FrP01Active_flg/2  "<VSRV_ISCHSC2FrP01Active_flg_ovrdflg>"
  Bus Selector1/1 -> Subsys VINP_ISCHSC2FrP01Active_flg/3  "<VSRV_ISCHSC2FrP01Active_flg_ovrdval>"
  Subsys VINP_ISCHSC2FrP01Active_flg/1 -> Bus Creator/7  "VINP_ISCHSC2FrP01Active_flg"
  [VINP_ISCMsgAlive_flg] -> Subsys VINP_ISCHSC2FrP01Active_flg/1, [MsgAlive_flgs]  "VINP_ISCMsgAlive_flg"
